simulink model "controller"  (R2022b)
settings: Solver=FixedStepAuto  StartTime=0.0  StopTime=10.0  FixedStep=1/100  RelTol=1e-3
undefined symbols (not defined in the file): MAX_SPEED_BACKWARD, MAX_SPEED_FORWARD, MAX_TORQUE, MAX_TORQUE_REVERSE, TransmissionState
libraries: slpidlib x1
settings Model: Creator=DAUIN-Win10  LastModifiedBy=Pietro
settings DebuggingCC: UnconnectedInputMsg=warning  UnconnectedOutputMsg=warning  UnconnectedLineMsg=warning
settings ModelReferenceCC: EnableRefExpFcnMdlSchedulingChecks=on
settings RTWCC: DLArmComputeVersion=19.05

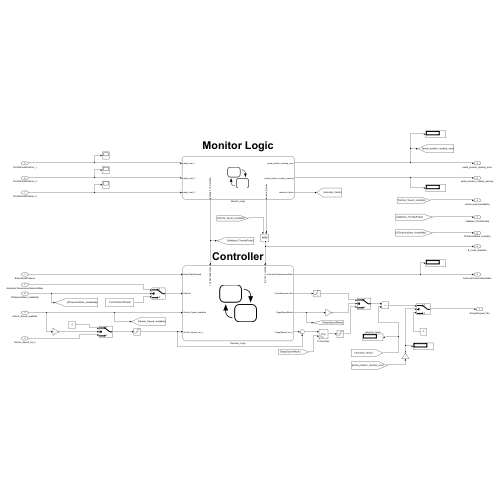
[thumbnail: Simulink's stored preview of the top-level diagram]
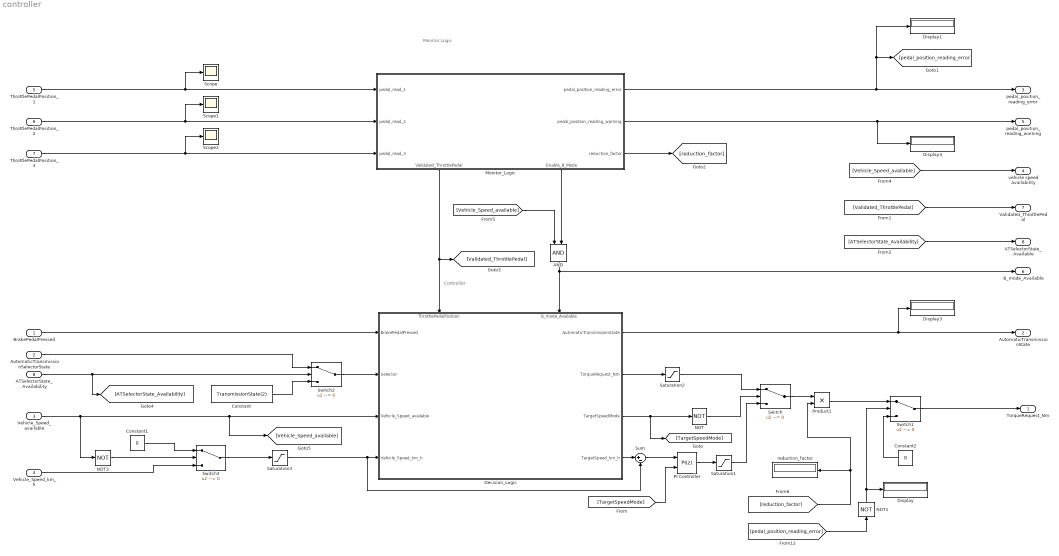
== system controller ==
  note: Monitor Logic
  note: Controller
  BrakePedalPressed : Inport  OutDataTypeStr=boolean
  AutomaticTransmissionSelectorState : Inport  Port=2  OutDataTypeStr=Enum: TransmissionState
  Vehicle_Speed_available : Inport  Port=3  OutDataTypeStr=boolean  Unit=km/h
  Vehicle_Speed_km_h : Inport  Port=4  OutDataTypeStr=single  Unit=km/h
  ThrottlePedalPosition_1 : Inport  Port=5  OutDataTypeStr=double
  ThrottlePedalPosition_2 : Inport  Port=6  OutDataTypeStr=double
  ThrottlePedalPosition_3 : Inport  Port=7  OutDataTypeStr=double
  ATSelectorState_Availability : Inport  Port=8  OutDataTypeStr=boolean
  AND : Logic  AllPortsSameDT=off  OutDataTypeStr=boolean
  Constant : Constant  Value=TransmissionState(2)
  Constant1 : Constant  Value=0  OutDataTypeStr=single
  Constant2 : Constant  Value=0  OutDataTypeStr=single
  Decision_Logic : Stateflow chart  TreatAsAtomicUnit=on
      settings: PortSchema="{\"entries\":[{\"content\":{\"sides\":[{\"content\":{\"connectorIds\":[\"In2\",\"In6\",\"In3\",\"In5\"]},\"type\":\"ConnectorPlacement.EquallySpacedRectSide\",\"uuid\":\"2f18118e-0843-4cb5-a956-6fbe9f973a93\"},{\"content\":{\"connectorIds\":[\"Out1\",\"Out2\",\"Out4\",\"Out3\"],\"side\":\"RIGHT\"},\"type\":\"ConnectorPlacement.EquallySpacedRectSide\",\"uuid\":\"8092894e-1a93-498e-82dc-1729ed135b0b\"},{\"content\":{\"connectorIds\":[\"In4\",\"In1\"],\"side\":\"TOP\"},\"type\":\"ConnectorPlacement.EquallySpacedRectSide\",\"uuid\":\"166517c2-1190-4c6d-a8f3-40e22d1b976e\"}]},\"type\":\"ConnectorPlacement.EquallySpacedConnector\",\"uuid\":\"ca5c1f38-53f7-468c-a97f-82447ab7a015\"}],\"packageUris\":[\"http://schema.mathworks.com/mf0/Connector/R2020b\"],\"version\":\"1.0\"}"
  Display{,1,3..4} (4 alike) : Display
  Monitor_Logic : Stateflow chart  TreatAsAtomicUnit=on
      settings: PortSchema="{\"entries\":[{\"content\":{\"sides\":[{\"content\":{\"connectorIds\":[\"In1\",\"In2\",\"In3\"]},\"type\":\"ConnectorPlacement.EquallySpacedRectSide\",\"uuid\":\"7e8062ab-7569-4291-8a74-652e83b32fc9\"},{\"content\":{\"connectorIds\":[\"Out1\",\"Out4\",\"Out5\"],\"side\":\"RIGHT\"},\"type\":\"ConnectorPlacement.EquallySpacedRectSide\",\"uuid\":\"87055ce6-60fb-4f5d-a4ce-509dd03ecabb\"},{\"content\":{\"connectorIds\":[],\"side\":\"TOP\"},\"type\":\"ConnectorPlacement.EquallySpacedRectSide\",\"uuid\":\"664d0b31-195e-4c3a-800d-28edce825c84\"},{\"content\":{\"connectorIds\":[\"Out3\",\"Out2\"],\"side\":\"BOTTOM\"},\"type\":\"ConnectorPlacement.EquallySpacedRectSide\",\"uuid\":\"dba6af62-ac30-49a2-a268-36ec45fb9dc4\"}]},\"type\":\"ConnectorPlacement.EquallySpacedConnector\",\"uuid\":\"f578971b-a210-44ee-957a-32c0f6c1d097\"}],\"packageUris\":[\"http://schema.mathworks.com/mf0/Connector/R2020b\"],\"version\":\"1.0\"}"
  NOT : Logic  Operator=NOT  IconShape=distinctive  AllPortsSameDT=off  OutDataTypeStr=boolean
  NOT1 : Logic  Operator=NOT  IconShape=distinctive  AllPortsSameDT=off  OutDataTypeStr=boolean
  NOT3 : Logic  Operator=NOT  IconShape=distinctive  AllPortsSameDT=off  OutDataTypeStr=boolean
  PI Controller : slpidlib/PID Controller  Controller=PI  Form=Parallel  TimeDomain=Discrete-time  UseExternalTs=on  SampleTime=-1  IntegratorMethod=Forward Euler  FilterMethod=Forward Euler  ControllerParametersSource=internal  P=100  I=0.1  UseKiTs=off  D=1  N=100  UseFilter=on  TunerSelectOption=Transfer Function Based (PID Tuner App)  InitialConditionSource=internal  InitialConditionForIntegrator=0  InitialConditionForFilter=0  DifferentiatorICPrevScaledInput=0  ExternalReset=none  TrackingMode=off  Kt=1  LimitOutput=off  SatLimitsSource=internal  UpperSaturationLimit=inf  LowerSaturationLimit=-inf  LinearizeAsGain=on  AntiWindupMode=none  Kb=1  LimitIntegrator=off  UpperIntegratorSaturationLimit=inf  LowerIntegratorSaturationLimit=-inf  POutMin=[]  POutMax=[]  IOutMin=[]  IOutMax=[]  DOutMin=[]  DOutMax=[]  NOutMin=[]  NOutMax=[]  SumOutMin=[]  SumOutMax=[]  SaturationOutMin=[]  SaturationOutMax=[]  PParamMin=[]  PParamMax=[]  IParamMin=[]  IParamMax=[]  DParamMin=[]  DParamMax=[]  NParamMin=[]  NParamMax=[]  KbParamMin=[]  KbParamMax=[]  KtParamMin=[]  KtParamMax=[]  KbOutMin=[]  KbOutMax=[]  KtOutMin=[]  KtOutMax=[]  IntegratorOutMin=[]  IntegratorOutMax=[]  FilterOutMin=[]  FilterOutMax=[]  SumI1OutMin=[]  SumI1OutMax=[]  SumI2OutMin=[]  SumI2OutMax=[]  SumI3OutMin=[]  SumI3OutMax=[]  SumI4OutMin=[]  SumI4OutMax=[]  SumDOutMin=[]  SumDOutMax=[]  DifferentiatorOutMin=[]  DifferentiatorOutMax=[]  FilterDiffOutCoefMin=[]  FilterDiffOutCoefMax=[]  ReciprocalOutMin=[]  ReciprocalOutMax=[]  SumDenOutMin=[]  SumDenOutMax=[]  SumNumOutMin=[]  SumNumOutMax=[]  DivideOutMin=[]  DivideOutMax=[]  UdiffTsProdOutMin=[]  UdiffTsProdOutMax=[]  NTsProdOutMin=[]  NTsProdOutMax=[]  UintegralTsProdOutMin=[]  UintegralTsProdOutMax=[]  UngainTsProdOutMin=[]  UngainTsProdOutMax=[]  ClampingZeroOutDataTypeStr=Inherit: Inherit via back propagation  ClampingZeroOutMin=[]  ClampingZeroOutMax=[]  FilterDenConstantOutDataTypeStr=Inherit: Inherit via back propagation  FilterDenConstantOutMin=[]  FilterDenConstantOutMax=[]  PCopyOutDataTypeStr=Inherit: Inherit via back propagation  PCopyOutMin=[]  PCopyOutMax=[]  NCopyOutDataTypeStr=Inherit: Inherit via back propagation  NCopyOutMin=[]  NCopyOutMax=[]  IntegratorContinuousStateAttributes=''  IntegratorStateMustResolveToSignalObject=off  IntegratorRTWStateStorageClass=Auto  FilterContinuousStateAttributes=''  FilterStateMustResolveToSignalObject=off  FilterRTWStateStorageClass=Auto  ParallelPVariant=InternalParameters  IdealPVariant=Disabled  IVariant=InternalParameters  DVariant=Disabled  IntegratorVariant=Discrete  SatVariant=Disabled  AWVariant=Passthrough  PCopyVariant=Disabled  TRVariant=Disabled  FdbkBlocksVariant=Forward  IdealPFdbkVariant=Disabled  SatFdbkVariant=Disabled  DerivativeFilterVariant=Disabled  NVariant=Disabled  NCopyVariant=Disabled_SignalSpec  FilterICVariant=Disabled  IntegratorICVariant=InternalICs  ExternalResetVariant=Disabled  TRSumVariant=Passthrough  SumFdbkVariant=Disabled  SumVariant=Sum_PI  TsampFilterVariant=InternalTs  TsampNgainVariant=Passthrough  TsampIntegralVariant=ExternalTs  ExternalSaturationOutDataTypeStr=Inherit: Same as second input
  Product1 : Product
  Saturation1 : Saturate  UpperLimit=MAX_TORQUE  LowerLimit=-MAX_TORQUE_REVERSE
  Saturation2 : Saturate  UpperLimit=MAX_TORQUE  LowerLimit=-MAX_TORQUE
  Saturation3 : Saturate  UpperLimit=MAX_SPEED_FORWARD  LowerLimit=-MAX_SPEED_BACKWARD  OutDataTypeStr=double
  Scope : Scope
  Scope1 : Scope
  Scope2 : Scope
  Sum : Sum  Inputs=|+-
  Switch{,1..3} (4 alike) : Switch  Criteria=u2 ~= 0  SaturateOnIntegerOverflow=off  InputSameDT=off
  reduction_factor : Display
  TorqueRequest_Nm : Outport  OutDataTypeStr=single  Unit=N*m
  AutomaticTransmissionState : Outport  Port=2  OutDataTypeStr=Enum: TransmissionState
  pedal_position_reading_error : Outport  Port=3  OutDataTypeStr=boolean
  vehicle speed availability : Outport  Port=4  OutDataTypeStr=boolean
  pedal_position_reading_warning : Outport  Port=5  OutDataTypeStr=boolean
  B_mode_Available : Outport  Port=6  OutDataTypeStr=boolean
  Validated_ThrottlePedal : Outport  Port=7  OutDataTypeStr=double
  ATSelectorState_Available : Outport  Port=8  OutDataTypeStr=boolean
  wires:
  BrakePedalPressed/1 -> Decision_Logic/2(BrakePedalPressed)
  Decision_Logic/2(TorqueRequest_Nm) -> Saturation2/1
  Decision_Logic/4(TargetSpeedMode) -> [TargetSpeedMode], NOT/1
  Saturation2/1 -> Switch/1
  NOT/1 -> Switch/2
  Decision_Logic/3(TargetSpeed_km_h) -> Sum/1
  PI Controller/1 -> Saturation1/1
  Saturation1/1 -> Switch/3
  Sum/1 -> PI Controller/1
  [TargetSpeedMode] -> PI Controller/2
  Saturation3/1 -> Sum/2, Decision_Logic/5(Vehicle_Speed_km_h)
  Switch1/1 -> TorqueRequest_Nm/1
  NOT1/1 -> Display/1, Switch1/2
  Constant2/1 -> Switch1/3
  Decision_Logic/1(AutomaticTransmissionState) -> AutomaticTransmissionState/1, Display3/1
  [pedal_position_reading_error] -> NOT1/1
  Monitor_Logic/3(Validated_ThrottlePedal) -> [Validated_ThrottlePedal], Decision_Logic/4(ThrottlePedalPosition)
  Switch3/1 -> Saturation3/1
  Vehicle_Speed_available/1 -> NOT3/1, [Vehicle_Speed_available], Decision_Logic/3(Vehicle_Speed_available)
  AND/1 -> Decision_Logic/1(B_mode_Available), B_mode_Available/1
  Monitor_Logic/2(Enable_B_Mode) -> AND/2
  [Vehicle_Speed_available] -> AND/1
  [Vehicle_Speed_available] -> vehicle speed availability/1
  Monitor_Logic/1(pedal_position_reading_error) -> [pedal_position_reading_error], Display1/1, pedal_position_reading_error/1
  Monitor_Logic/4(pedal_position_reading_warning) -> pedal_position_reading_warning/1, Display4/1
  Monitor_Logic/5(reduction_factor) -> [reduction_factor]
  Switch/1 -> Product1/1
  [reduction_factor] -> Product1/2, reduction_factor/1
  Product1/1 -> Switch1/1
  ThrottlePedalPosition_3/1 -> Scope2/1, Monitor_Logic/3(pedal_read_3)
  ThrottlePedalPosition_2/1 -> Scope1/1, Monitor_Logic/2(pedal_read_2)
  ThrottlePedalPosition_1/1 -> Scope/1, Monitor_Logic/1(pedal_read_1)
  [Validated_ThrottlePedal] -> Validated_ThrottlePedal/1
  ATSelectorState_Availability/1 -> [ATSelectorState_Availability], Switch2/2
  Switch2/1 -> Decision_Logic/6(Selector)
  [ATSelectorState_Availability] -> ATSelectorState_Available/1
  AutomaticTransmissionSelectorState/1 -> Switch2/1
  Constant/1 -> Switch2/3
  Vehicle_Speed_km_h/1 -> Switch3/3
  Constant1/1 -> Switch3/1
  NOT3/1 -> Switch3/2

== stateflow chart controller/Monitor_Logic ==
  state Fault_mode
    entry:
    Enable_B_Mode = false
    reduction_factor = 0.7
    state pedal_read_1_wrong
      entry:
      pedal_position_reading_warning = true
      during:
      Validated_ThrottlePedal =...
      (pedal_read_2+pedal_read_3)/2
    state pedal_read_3_wrong
      entry:
      pedal_position_reading_warning = true
      during:
      Validated_ThrottlePedal =...
      (pedal_read_2+pedal_read_1)/2
    state pedal_read_2_wrong
      entry:
      pedal_position_reading_warning = true
      during:
      Validated_ThrottlePedal =...
      (pedal_read_1+pedal_read_3)/2
    state No_pedal_read
      entry:
      pedal_position_reading_error = true;
    (default) -> (junction 66)
    (junction 66) -> pedal_read_3_wrong [order 2] : [Flag == 3]
    (junction 66) -> pedal_read_1_wrong [order 5]
    (junction 66) -> pedal_read_2_wrong [order 4] : [Flag == 2]
    (junction 66) -> pedal_read_1_wrong [order 1] : [Flag == 1]
    (junction 66) -> No_pedal_read [order 3] : [Flag == 4]
    pedal_read_2_wrong -> No_pedal_read : [Flag == 4]
    pedal_read_3_wrong -> No_pedal_read : [Flag == 4]
    pedal_read_1_wrong -> No_pedal_read : [Flag == 4]
  state Normal_mode
    entry:
    pedal_position_reading_warning = false
    pedal_position_reading_error=false
    Enable_B_Mode = true
    Flag = -1
    reduction_factor=1
    during:
    Validated_ThrottlePedal = (pedal_read_1 + pedal_read_2 + pedal_read_3)/3
  Fault_mode -> Fault_mode [order 2] : [abs(pedal_read_1-pedal_read_2)  >= 0.01 && abs(pedal_read_2-pedal_read_3)  >= 0.01...
      |  && abs(pedal_read_1-pedal_read_3) >= 0.01 && Flag ~= 4]{Flag = 4}
  (default) -> Normal_mode
  Normal_mode -> Fault_mode [order 2] : [abs(pedal_read_1-pedal_read_2)  >= 0.01 &&...
      |  abs(pedal_read_1-pedal_read_3) >= 0.01 &&...
      |  abs(pedal_read_2-pedal_read_3) < 0.01]{Flag = 1}
  Normal_mode -> Fault_mode [order 3] : [abs(pedal_read_1-pedal_read_2)  >= 0.01 &&...
      |  abs(pedal_read_2-pedal_read_3) >= 0.01 &&...
      |  abs(pedal_read_1-pedal_read_3) < 0.01]{Flag = 2}
  Normal_mode -> Fault_mode [order 4] : [abs(pedal_read_1-pedal_read_3)  >= 0.01 &&...
      |  abs(pedal_read_2-pedal_read_3) >= 0.01 &&...
      |  abs(pedal_read_1-pedal_read_2) < 0.01]{Flag = 3}
  Normal_mode -> Fault_mode [order 1] : [abs(pedal_read_1-pedal_read_2)  >= 0.01 && abs(pedal_read_2-pedal_read_3)  >= 0.01...
      |  && abs(pedal_read_1-pedal_read_3) >= 0.01]{Flag = 4}
  Fault_mode -> Normal_mode [order 1] : [ duration(abs(pedal_read_1-pedal_read_2)  < 0.01 &&...
      |   abs(pedal_read_2-pedal_read_3)  < 0.01) > 20 ]
  data: pedal_position_reading_error output; Enable_B_Mode output; pedal_read_1 input; pedal_read_2 input; pedal_read_3 input; Validated_ThrottlePedal output; Flag local; pedal_position_reading_warning output; reduction_factor output

== stateflow chart controller/Decision_Logic ==
  state Brake_mode
    entry:
    AutomaticTransmissionState = TransmissionState(4);
    state Car_stopped
      entry:
      TargetSpeed_km_h = 0;
      TargetSpeedMode = 1;
      exit:
      TargetSpeedMode = 0;
      TorqueRequest_Nm = 0;
    state Acceleration
      during:
      TorqueRequest_Nm = MAX_TORQUE*...
      3/2*(ThrottlePedalPosition-1/3);
    state Regenerative_Breaking
      during:
      TorqueRequest_Nm = -MAX_TORQUE*...
      (1-3*ThrottlePedalPosition);
    (default) -> (junction 178)
    (junction 178) -> Car_stopped [order 2] : [abs(Vehicle_Speed_km_h) <= 0.5 &&...
        |  ThrottlePedalPosition <= 1/3 ]
    (junction 178) -> Acceleration [order 3]
    (junction 178) -> Acceleration [order 1] : [ThrottlePedalPosition > 1/3]
    Car_stopped -> Acceleration : [ThrottlePedalPosition > 1/3]
    Regenerative_Breaking -> Car_stopped [order 2] : [Vehicle_Speed_km_h <= 0.5]
    Acceleration -> Regenerative_Breaking : [ThrottlePedalPosition <= 1/3 ]
    Regenerative_Breaking -> Acceleration [order 1] : [ThrottlePedalPosition > 1/3 ]
  state Brake_Pedal
    state Released
      entry:
      TargetSpeedMode = 1;
      exit:
      TargetSpeedMode = 0;
    state Pressed
      entry:
      TorqueRequest_Nm = 0;
    (default) -> Pressed
    Pressed -> Released : [BrakePedalPressed == false && ...
        | abs(Vehicle_Speed_km_h) <= 0.5 && ...
        | Vehicle_Speed_available==true]
    Released -> Pressed : [BrakePedalPressed == true]
  note: Park(0)
      | Reverse(1)
      | Neutral(2)
      | Drive(3)
      | Brake(4)
  state Drive_mode
    entry:
    AutomaticTransmissionState = TransmissionState(3);
    during:
    TorqueRequest_Nm = MAX_TORQUE*ThrottlePedalPosition;
  state Neutral_mode
    entry:
    AutomaticTransmissionState = TransmissionState(2);
    during:
    TorqueRequest_Nm = 0;
  state Park_mode
    entry:
    AutomaticTransmissionState = TransmissionState(0);
    TargetSpeedMode = 0;
    TargetSpeed_km_h = 0;
    during:
    TorqueRequest_Nm = 0;
  state Reverse_mode
    entry:
    AutomaticTransmissionState = TransmissionState(1);
    during:
    TorqueRequest_Nm = -1*MAX_TORQUE_REVERSE*ThrottlePedalPosition;
  (junction 220) -> Brake_mode
  Brake_Pedal -> (junction 220) [order 2] : [AutomaticTransmissionState == 4 &&...
      |  ThrottlePedalPosition > 1/3 && BrakePedalPressed == false && ...
      | B_mode_Available==true]
  Brake_mode -> Brake_Pedal [order 2] : [BrakePedalPressed == true]
      | {TargetSpeed_km_h = 5}
  (junction 218) -> Brake_Pedal
  Brake_Pedal -> (junction 216) [order 3] : [((Selector <= 3 || B_mode_Available==false) && ...
      |  AutomaticTransmissionState == 4)...
      | || (AutomaticTransmissionState == 3 &&...
      |  ThrottlePedalPosition > 0 && BrakePedalPressed == false )]
  Brake_Pedal -> (junction 214) [order 1] : [(Selector <= 2 && AutomaticTransmissionState == 3) ||...
      | (Selector ~= 1 && AutomaticTransmissionState == 1)]
  Brake_Pedal -> (junction 212) [order 4] : [AutomaticTransmissionState == 1 &&...
      |  ThrottlePedalPosition > 0 && BrakePedalPressed == false]
  (junction 210) -> Brake_Pedal
  Brake_mode -> Drive_mode [order 1] : [Selector ~= 4 || ...
      | B_mode_Available==false]
  Drive_mode -> Brake_mode [order 2] : [Selector == 4 && (ThrottlePedalPosition > 1/3  || ...
      | abs(Vehicle_Speed_km_h) <= 0.5) &&...
      | B_mode_Available==true]
  Drive_mode -> (junction 218) [order 3] : [BrakePedalPressed == true]
      | {TargetSpeed_km_h = 5}
  (junction 216) -> Drive_mode
  Drive_mode -> Neutral_mode [order 1] : [Selector <= 2]
  Neutral_mode -> Drive_mode [order 1] : [Selector >= 3 && Vehicle_Speed_km_h > -5 && BrakePedalPressed]
  (default) -> Park_mode
  (junction 214) -> Neutral_mode
  Park_mode -> Neutral_mode : [Selector ~= 0 && BrakePedalPressed]
  Neutral_mode -> Park_mode [order 3] : [Selector == 0 && abs(Vehicle_Speed_km_h) < 5 ...
      | && BrakePedalPressed]
  Reverse_mode -> Neutral_mode [order 1] : [Selector ~= 1]
  Neutral_mode -> Reverse_mode [order 2] : [Selector == 1 && Vehicle_Speed_km_h < 5 && BrakePedalPressed]
  (junction 212) -> Reverse_mode
  Reverse_mode -> (junction 210) [order 2] : [BrakePedalPressed == true]
      | {TargetSpeed_km_h = -5}
  data: B_mode_Available input; BrakePedalPressed input; Vehicle_Speed_available input; ThrottlePedalPosition input; Vehicle_Speed_km_h input; AutomaticTransmissionState output; TorqueRequest_Nm output; MAX_TORQUE parameter; MAX_TORQUE_REVERSE parameter; TargetSpeed_km_h output; TargetSpeedMode output; Selector input
